simulink model "AbstractCombustionEngineCar_1_KHUSHI (3)"  (R2025a)
settings: Solver=FixedStepAuto  StartTime=0.0  StopTime=1200  FixedStep=0.001  MaxStep=0.001  RelTol=1e-3  AbsTol=1e-3
PreLoadFcn:
  | AbstractCombustionEngineCarSetup
libraries: fl_lib x18, nesl_utility x13, sdl_lib x5
CloseFcn:
  | try,close(h1_AbstractCombustionEngineCar),end
  | clear h1_AbstractCombustionEngineCar
  | 
  | try,close(h2_AbstractCombustionEngineCar),end
  | clear h2_AbstractCombustionEngineCar
  | 
  | try,close(h3_AbstractCombustionEngineCar),end
  | clear h3_AbstractCombustionEngineCar
  | 
  | clear tout_AbstractCombustionEngineCar
  | clear logsout_AbstractCombustionEngineCar
  | clear simlog_AbstractCombustionEngineCar
  | 
  | clear AbstractCombustionEngineCarInputplot
  | clear AbstractCombustionEngineCar_Signals
  | clear AbstractCombustionEngineCar_Bus
settings Model: Creator=The MathWorks, Inc.  LastModifiedBy=rajde
settings SolverCC: AutoScaleAbsTol=off  DaesscMode=Balanced  MaxZcPerStep=1.0
settings DataIOCC: SaveOutput=off  DSMLogging=off  ReturnWorkspaceOutputs=off  TimeSaveName=tout_AbstractCombustionEngineCar  SignalLoggingName=logsout_AbstractCombustionEngineCar  ReturnWorkspaceOutputsName=out_AbstractCombustionEngineCar
settings OptimizationCC: ReuseModelBlockBuffer=off
settings ModelReferenceCC: EnableRefExpFcnMdlSchedulingChecks=on
settings RTWCC: GPUComputeCapability=3.5
settings SimscapeCC: SimscapeLogType=all  SimscapeLogSimulationStatistics=on  SimscapeLogName=simlog_AbstractCombustionEngineCar  SimscapeLogLimitData=off

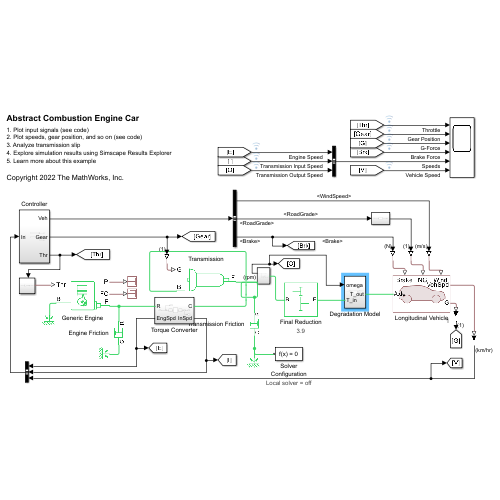
[thumbnail: Simulink's stored preview of the top-level diagram]
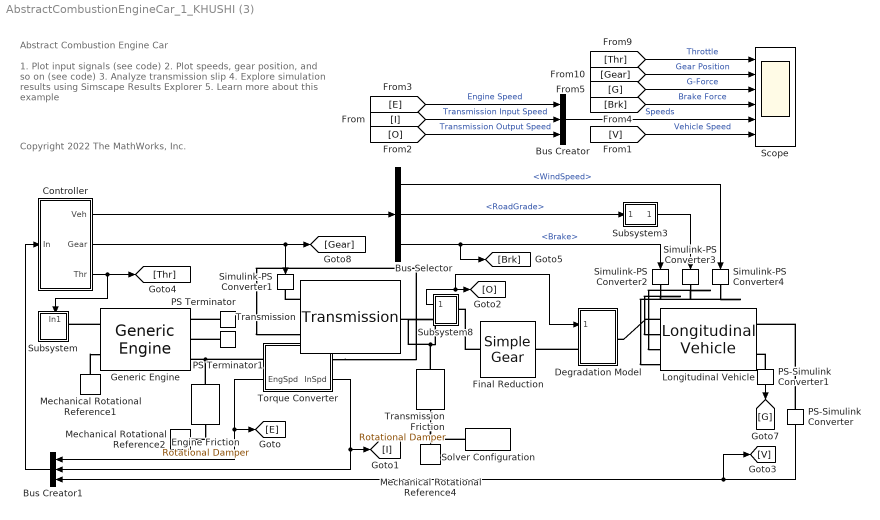
== system AbstractCombustionEngineCar_1_KHUSHI (3) ==
  note: 1. Plot input signals (see code)
      | 2. Plot speeds, gear position, and so on (see code)
      | 3. Analyze transmission slip
      | 4. Explore simulation results using Simscape Results Explorer
      | 5. Learn more about this example
  note: Abstract Combustion Engine Car
  note: Copyright 2022 The MathWorks, Inc.
  Bus Creator : BusCreator  Inputs=3
  Bus Creator1 : BusCreator  Inputs=3
  Bus Selector : BusSelector  OutputSignals=WindSpeed,RoadGrade,Brake
  Controller : Subsystem
  Degradation Model : Subsystem
  Engine Friction : fl_lib/Mechanical/Rotational Elements/Rotational Damper  D=0.01 N*m/rpm  w_specify=off  w_priority=None  w=0 rad/s  w_nominal_specify=off  w_nominal_value=1  w_nominal_unit=rad/s  t_specify=off  t_priority=None  t=0 N*m  t_nominal_specify=off  t_nominal_value=1  t_nominal_unit=N*m
  Final Reduction : sdl_lib/Gears/Simple Gear  ratio=3.9  rotation_direction=sdl.enum.shaftOutputDirection.same  friction_model=sdl.enum.gear_efficiencies_load.off  T_noload=0.1 N*m  T_nom=5 N*m  efficiency_nom=0.8  efficiency=0.8  temperature_TLU=[280, 300, 320] K  load_TLU=[1, 5, 10] N*m  efficiency_TLU=[.95, .9, .85]  efficiency_TLU2=[.85, .8, .75; .95, .9, .85; .85, .8, .7]  w_thr=0.01 rad/s  pwr_thr=0.001 W  enable_backlash=false  hardstop_model=simscape.enum.hardstop.smooth  backlash_distance=1e-3 mm  r_base=0.1 m  transition=1e-4 mm  backlash_stiffness=1e7 N/m  backlash_damping=1e6 N*s/m  coeff_rest=0  v_tol=0.001 m/s  f_tol=0 N  mu_visc=[0, 0] N*m*s/rad  thermal_mass=50 J/K  temperature_specify=off  temperature_priority=High  temperature=300 K  temperature_nominal_specify=off  temperature_nominal_value=1  temperature_nominal_unit=K  x_backlash_specify=off  x_backlash_priority=None  x_backlash=0 mm  x_backlash_nominal_specify=off  x_backlash_nominal_value=1  x_backlash_nominal_unit=mm  f_hardstop_specify=off  f_hardstop_priority=None  f_hardstop=0 N  f_hardstop_nominal_specify=off  f_hardstop_nominal_value=1  f_hardstop_nominal_unit=N  v_backlash_specify=off  v_backlash_priority=None  v_backlash=0 m/s  v_backlash_nominal_specify=off  v_backlash_nominal_value=1  v_backlash_nominal_unit=m/s
      settings: AttributesFormatString=%<ratio>
  Generic Engine : sdl_lib/Engines & Motors/Generic Engine  input_type=sdl.enum.GenericEngineInputType.NormalizedThrottle  model_parameterization=sdl.enum.engineParameterization.polynomial  engine_type=sdl.enum.engineType.SI  Trq_max=380 N*m  w_Trq_max=4300 rpm  P_max=150 kW  w_P_max=4500 rpm  w_max=6000 rpm  w_min=500 rpm  w_tab=[500, 1000, 2000, 3000, 4000, 5000, 6000, 7000] rpm  trq_tab=[380, 380, 380, 380, 350, 280, 200, 80] N*m  pwr_tab=[20, 40, 78, 120, 145, 148, 125, 60] kW  interp_method=simscape.enum.interpolation.linear  w_thr=100 rpm  model_inertia=sdl.enum.model_inertia.on  inertia=0.02 kg*m^2  initial_velocity=800 rpm  model_time_constant=sdl.enum.lagOffOn.off  time_constant=0.2 s  initial_normalized_throttle=0  fc_model=sdl.enum.fuel_consumption_model.FuelOff  fc_per_rev=25 mg/rev  fc_w_tab=[1000, 2000, 3000, 4000, 5000, 6000] rpm  fc_trq_tab=[0, 80, 160, 200, 240, 320, 360, 400] N*m  fc_tab=[.5, .9, 1.4, 1.6, 1.9, 2.7, 3.4, 4.4; 1, 1.7, 2.7, 3.1, 3.6, 5, 6, 7.4; 1.4, 2.7, 4, 4.8, 5.6, 7.5, 8.5, 10.5; 2, 3.6, 5.8, 6.7, 8, 10.4, 11.7, 13.3; 2.5, 4.8, 7.9, 9.4, 10.8, 14, 16.2, 18.6; 3.1, 6, 10.3, 11.9, 13.8, 18.4, 22, 26.5] g/s  bmep_tab=[0, 250, 500, 625, 750, 1000, 1150, 1250] kPa  bsfc_tab=[410, 380, 300, 280, 270, 290, 320, 380; 410, 370, 290, 270, 260, 270, 285, 320; 415, 380, 290, 275, 265, 270, 270, 300; 420, 390, 310, 290, 285, 280, 280, 285; 430, 410, 340, 320, 310, 300, 310, 320; 450, 430, 370, 340, 330, 330, 350, 380] g/(hr*kW)  fc_interp_method=simscape.enum.interpolation.linear  displaced_volume=400 cm^3  rev_per_cycle=2  idle_speed=simscape.enum.onoff.on  idle_speed_reference=800 rpm  tau_controller=0.1 s  idle_w_thr=10 rpm  redline=simscape.enum.onoff.off  redline_speed=7500 rpm  tau_redline=1 s  redline_w_thr=1 rpm
      settings: InternalSimscapePortConfiguration="{\"Bottom\":[],\"Left\":[{\"id\":\"ThrNorm\",\"label\":\"Thr\",\"type\":\"input\"},{\"id\":\"B\",\"label\":\"B\",\"type\":\"foundation.mechanical.rotational.rotational\"}],\"Right\":[{\"id\":\"P\",\"label\":\"P\",\"type\":\"output\"},{\"id\":\"FC\",\"label\":\"FC\",\"type\":\"output\"},{\"id\":\"F\",\"label\":\"F\",\"type\":\"foundation.mechanical.rotational.rotational\"}],\"Top\":[]}"
  Longitudinal Vehicle : sdl_lib/Tires & Vehicles/Longitudinal Vehicle  vehParamType=sdl.enum.VehicleParameterizationType.Large  M_vehicle=1200 kg  R_tireroll=0.3 m  C_tireroll=0.0136  C_airdrag=0.31  A_front=2.3 m^2  A_rl=120 N  B_rl=1.8 N*s/m  C_rl=0.389 N*s^2/m^2  g=9.81 m/s^2  V_1=0.3 m/s  w_1=0.01 rad/s  ShowBrakeIn=simscape.enum.onoff.on  ShowSlopeIn=simscape.enum.onoff.on  SlopeInputType=sdl.enum.VehicleLongitudinalRoadSlopeInputType.Grade  ShowWindIn=simscape.enum.onoff.on  ShowGOut=simscape.enum.onoff.on  air_density=1.184 kg/m^3  V_x_specify=off  V_x_priority=High  V_x=0 km/hr  V_x_nominal_specify=off  V_x_nominal_value=1  V_x_nominal_unit=m/s  trq_specify=off  trq_priority=None  trq=0 N*m  trq_nominal_specify=off  trq_nominal_value=1  trq_nominal_unit=N*m  w_specify=off  w_priority=None  w=0 rad/s  w_nominal_specify=off  w_nominal_value=1  w_nominal_unit=rad/s
      settings: InternalSimscapePortConfiguration="{\"Bottom\":[],\"Left\":[{\"id\":\"Axle\",\"label\":\"Axle\",\"type\":\"foundation.mechanical.rotational.rotational\"}],\"Right\":[{\"id\":\"v_out\",\"label\":\"VehSpd\",\"type\":\"output\"},{\"id\":\"G_out\",\"label\":\"G\",\"type\":\"output\"}],\"Top\":[{\"id\":\"brkF\",\"label\":\"Brake\",\"type\":\"input\"},{\"id\":\"grade_norm\",\"label\":\"NG\",\"type\":\"input\"},{\"id\":\"V_wind\",\"label\":\"Wind\",\"type\":\"input\"}]}"
  Mechanical Rotational Reference1 : fl_lib/Mechanical/Rotational Elements/Mechanical Rotational Reference
  Mechanical Rotational Reference2 : fl_lib/Mechanical/Rotational Elements/Mechanical Rotational Reference
  Mechanical Rotational Reference4 : fl_lib/Mechanical/Rotational Elements/Mechanical Rotational Reference
  PS Terminator : fl_lib/Physical Signals/Sinks/PS Terminator
  PS Terminator1 : fl_lib/Physical Signals/Sinks/PS Terminator
  PS-Simulink Converter : nesl_utility/PS-Simulink Converter  PhysicalDomain=network_engine_domain  SubClassName=ps_output  LeftPortType=input  RightPortType=output  PseudoPeriodic=off  Frequencies=[]  VectorFormat=inherit  Unit=km/hr  AffineConversion=off
  PS-Simulink Converter1 : nesl_utility/PS-Simulink Converter  PhysicalDomain=network_engine_domain  SubClassName=ps_output  LeftPortType=input  RightPortType=output  PseudoPeriodic=off  Frequencies=[]  VectorFormat=inherit  Unit=1  AffineConversion=off
  Scope : Scope  NumInputPorts=6
      settings: ActiveDisplayYMinimum=-11.25  ActiveDisplayYMaximum=101.25
  Simulink-PS Converter1 : nesl_utility/Simulink-PS Converter  PhysicalDomain=network_engine_domain  SubClassName=ps_input  LeftPortType=input  RightPortType=output  PseudoPeriodic=off  Frequencies=[]  NoiseDistribution=none  NoiseParameters=[]  Unit=1  AffineConversion=off  FilteringAndDerivatives=provide  SimscapeFilterOrder=1  InputFilterTimeConstant=0.001  UdotUserProvided=0
  Simulink-PS Converter2 : nesl_utility/Simulink-PS Converter  PhysicalDomain=network_engine_domain  SubClassName=ps_input  LeftPortType=input  RightPortType=output  PseudoPeriodic=off  Frequencies=[]  NoiseDistribution=none  NoiseParameters=[]  Unit=N  AffineConversion=off  FilteringAndDerivatives=provide  SimscapeFilterOrder=1  InputFilterTimeConstant=0.001  UdotUserProvided=0
  Simulink-PS Converter3 : nesl_utility/Simulink-PS Converter  PhysicalDomain=network_engine_domain  SubClassName=ps_input  LeftPortType=input  RightPortType=output  PseudoPeriodic=off  Frequencies=[]  NoiseDistribution=none  NoiseParameters=[]  Unit=1  AffineConversion=off  FilteringAndDerivatives=provide  SimscapeFilterOrder=1  InputFilterTimeConstant=0.001  UdotUserProvided=0
  Simulink-PS Converter4 : nesl_utility/Simulink-PS Converter  PhysicalDomain=network_engine_domain  SubClassName=ps_input  LeftPortType=input  RightPortType=output  PseudoPeriodic=off  Frequencies=[]  NoiseDistribution=none  NoiseParameters=[]  Unit=m/s  AffineConversion=off  FilteringAndDerivatives=provide  SimscapeFilterOrder=1  InputFilterTimeConstant=0.001  UdotUserProvided=0
  Solver Configuration : nesl_utility/Solver Configuration  PhysicalDomain=network_engine_domain  SubClassName=solver  LeftPortType=input  RightPortType=generic  Tones=[]  Harmonics=[]  SimulateNoise=off  Profile=off  UseLocalSampling=off  EnableSwitchedLinearOptims=on  FrequencyDomain=off  UseCCode=off  RelTol=0.001  AbsTol=0.001  MinStep=1e-09  ToWorkspace=off  RevertToSquareIcSolve=off  NumHomotopyIterations=100  PhasorMode=off  PhasorModeNumHarmonics=1  ConsistencySolver=NEWTON_XTOL_AFTER_FTOL  IndexReductionMethod=DerivativeReplacement  DoDC=off  ResidualTolerance=1e-09  ConsistencyTolSource=GLOBAL  ConsistencyAbsTol=0.001  ConsistencyRelTol=0.001  ConsistencyTolFactor=0.001  UseLocalSolver=off  LocalSolverChoice=NE_BACKWARD_EULER_ADVANCER  ResolveIndetEquations=on  FunctionEvalNumThread=1  LocalSolverSampleTime=0.001  DoFixedCost=off  MaxNonlinIter=3  MaxModeIter=2  ComputeImpulses=off  ImpulseIterations=2  LinearAlgebra=auto  LinearAlgebraNumThread=0  EquationFormulation=NE_TIME_EF  DelaysMemoryBudget=1024  AutomaticFiltering=on  FilteringTimeConstant=0.001  PartitionStorageMethod=AS_NEEDED  PartitionMemoryBudget=1024  PartitionMethod=ROBUST  MultibodyUseLocalSolver=off  MultibodyLocalSolverChoice=ODE1  MultibodyLocalSolverSampleTime=0.001
      settings: AttributesFormatString=Local solver = %<UseLocalSolver>
  Subsystem : Subsystem
      settings: PortSchema="{\"entries\":[{\"content\":{\"sides\":[{\"content\":{\"connectorIds\":[]},\"type\":\"ConnectorPlacement.EquallySpacedRectSide\",\"uuid\":\"38476285-4b1d-4cfe-b9ba-56388b6e142d\"},{\"content\":{\"connectorIds\":[\"RConn1\"],\"side\":\"RIGHT\"},\"type\":\"ConnectorPlacement.EquallySpacedRectSide\",\"uuid\":\"ba0e92dd-90b0-4ff2-bfbd-3d18e117ce00\"},{\"content\":{\"connectorIds\":[\"In1\"],\"side\":\"TOP\"},\"type\":\"ConnectorPlacement.EquallySpacedRectSide\",\"uuid\":\"d72bcda9-1129-409b-a624-7361223ab5f8\"}]},\"type\":\"ConnectorPlacement.EquallySpacedConnector\",\"uuid\":\"46949968-9b34-453f-a959-32b8a4fd4c57\"}],\"packageUris\":[\"http://schema.mathworks.com/mf0/Connector/R2020b\"],\"version\":\"1.0\"}"
  Subsystem3 : Subsystem
  Subsystem8 : Subsystem
      settings: PortSchema="{\"entries\":[{\"content\":{\"sides\":[{\"content\":{\"connectorIds\":[\"Out1\",\"LConn1\"]},\"type\":\"ConnectorPlacement.EquallySpacedRectSide\",\"uuid\":\"a87ce211-5ca3-4dba-a83b-da94e949f171\"},{\"content\":{\"connectorIds\":[\"RConn1\"],\"side\":\"RIGHT\"},\"type\":\"ConnectorPlacement.EquallySpacedRectSide\",\"uuid\":\"788867ba-271d-48ee-bf4b-70614e75db20\"},{\"content\":{\"connectorIds\":[],\"side\":\"TOP\"},\"type\":\"ConnectorPlacement.EquallySpacedRectSide\",\"uuid\":\"607020b5-dd3c-48e1-9492-c22d083697f7\"},{\"content\":{\"connectorIds\":[],\"side\":\"BOTTOM\"},\"type\":\"ConnectorPlacement.EquallySpacedRectSide\",\"uuid\":\"61462458-f4c7-4735-9817-1b1875f46976\"}]},\"type\":\"ConnectorPlacement.EquallySpacedConnector\",\"uuid\":\"473fa968-ffd5-4c8c-8204-df51e2cb909e\"}],\"packageUris\":[\"http://schema.mathworks.com/mf0/Connector/R2020b\"],\"version\":\"1.0\"}"
  Torque Converter : Subsystem
      settings: PortSchema="{\"entries\":[{\"content\":{\"sides\":[{\"content\":{\"connectorIds\":[\"LConn1\",\"Out2\"]},\"type\":\"ConnectorPlacement.EquallySpacedRectSide\",\"uuid\":\"617538e0-3440-487d-b133-1f4231421eb5\"},{\"content\":{\"connectorIds\":[\"RConn1\",\"Out1\"],\"side\":\"RIGHT\"},\"type\":\"ConnectorPlacement.EquallySpacedRectSide\",\"uuid\":\"0cc25c53-6bfd-4172-944f-9e7138ffc800\"},{\"content\":{\"connectorIds\":[],\"side\":\"TOP\"},\"type\":\"ConnectorPlacement.EquallySpacedRectSide\",\"uuid\":\"814870c3-fb4e-4999-b1ac-f0bc310280a4\"},{\"content\":{\"connectorIds\":[],\"side\":\"BOTTOM\"},\"type\":\"ConnectorPlacement.EquallySpacedRectSide\",\"uuid\":\"65ae3c81-05f8-4b99-bf66-538c9dc41f9a\"}]},\"type\":\"ConnectorPlacement.EquallySpacedConnector\",\"uuid\":\"f25e6ec4-4b55-4318-8ed3-0c35c2cb6893\"}],\"packageUris\":[\"http://schema.mathworks.com/mf0/Connector/R2020b\"],\"version\":\"1.0\"}"
  Transmission : sdl_lib/Gears/Transmission  gear_ratios=[2.3, 1.6, 1.2, 1, .8, .6]  reverse_ratio=-3  friction_model=sdl.enum.transmissionFriction.none  efficiency=0.95  efficiency_tlu=[.95, .95, .95, .95, .95, .95]  reverse_efficiency=0.90  pwr_thr=0.001 W  kp=3e5 N*m/rad  kv=3e4 N*m*s/rad  initial_torque=0 N*m  mu_visc=[0, 0] N*m*s/rad  t_friction=1000 N*m  t_locked=1000 N*m  shift_model=sdl.enum.transmissionShiftModel.instant  shift_time=200 ms  w_tol=0.001 rad/s  initial_state_locked=sdl.enum.initial_lock.locked  thermal_port=simscape.enum.thermaleffects.omit  thermal_mass=100 kJ/K  initial_temperature=300 K
      settings: InternalSimscapePortConfiguration="{\"Bottom\":[],\"Left\":[{\"id\":\"G\",\"label\":\"G\",\"type\":\"input\"},{\"id\":\"B\",\"label\":\"B\",\"type\":\"foundation.mechanical.rotational.rotational\"}],\"Right\":[{\"id\":\"F\",\"label\":\"F\",\"type\":\"foundation.mechanical.rotational.rotational\"}],\"Top\":[]}"
  Transmission Friction : fl_lib/Mechanical/Rotational Elements/Rotational Damper  D=0.001 N*m/rpm  w_specify=off  w_priority=None  w=0 rad/s  w_nominal_specify=off  w_nominal_value=1  w_nominal_unit=rad/s  t_specify=off  t_priority=None  t=0 N*m  t_nominal_specify=off  t_nominal_value=1  t_nominal_unit=N*m
  wires:
  Subsystem8/1(Spd) -> Degradation Model/1(omega), [O]
  [I] -> Bus Creator/2  "Transmission Input Speed"
  [O] -> Bus Creator/3  "Transmission Output Speed"
  [E] -> Bus Creator/1  "Engine Speed"
  Torque Converter/2(EngSpd) -> [E], Bus Creator1/1
  PS-Simulink Converter/1 -> Bus Creator1/3, [V]
  Bus Creator1/1 -> Controller/1(In)
  Controller/1(Veh) -> Bus Selector/1
  Torque Converter/1(InSpd) -> Bus Creator1/2, [I]
  [Thr] -> Scope/1  "Throttle"
  Bus Selector/3 -> [Brk], Simulink-PS Converter2/1  "<Brake>"
  Bus Selector/2 -> Subsystem3/1(In1)  "<RoadGrade>"
  Bus Selector/1 -> Simulink-PS Converter4/1  "<WindSpeed>"
  Subsystem3/1(Out1) -> Simulink-PS Converter3/1
  [V] -> Scope/6  "Vehicle Speed"
  Bus Creator/1 -> Scope/5  "Speeds"
  [G] -> Scope/3  "G-Force"
  Controller/3(Thr) -> [Thr], Subsystem/1(In1)
  Controller/2(Gear) -> Simulink-PS Converter1/1, [Gear]
  PS-Simulink Converter1/1 -> [G]
  [Brk] -> Scope/4  "Brake Force"
  [Gear] -> Scope/2  "Gear Position"
  connections:
  Torque Converter/LConn1 -- Engine Friction/LConn1 -- Generic Engine/RConn3
  Engine Friction/RConn1 -- Mechanical Rotational Reference2/LConn1
  Mechanical Rotational Reference1/LConn1 -- Generic Engine/LConn2
  Transmission Friction/LConn1 -- Transmission/RConn1 -- Subsystem8/LConn1
  Transmission/LConn1 -- Simulink-PS Converter1/RConn1
  Transmission Friction/RConn1 -- Solver Configuration/RConn1 -- Mechanical Rotational Reference4/LConn1
  PS-Simulink Converter/LConn1 -- Longitudinal Vehicle/RConn1
  Simulink-PS Converter3/RConn1 -- Longitudinal Vehicle/LConn3
  Simulink-PS Converter2/RConn1 -- Longitudinal Vehicle/LConn2
  Simulink-PS Converter4/RConn1 -- Longitudinal Vehicle/LConn4
  Torque Converter/RConn1 -- Transmission/LConn2
  Final Reduction/LConn1 -- Subsystem8/RConn1
  Generic Engine/LConn1 -- Subsystem/RConn1
  PS-Simulink Converter1/LConn1 -- Longitudinal Vehicle/RConn2
  PS Terminator/LConn1 -- Generic Engine/RConn1
  PS Terminator1/LConn1 -- Generic Engine/RConn2
  Degradation Model/LConn1 -- Final Reduction/RConn1
  Longitudinal Vehicle/LConn1 -- Degradation Model/RConn1

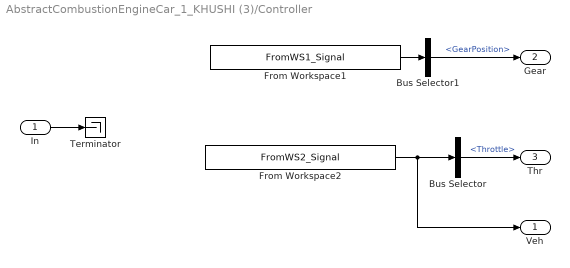
== system AbstractCombustionEngineCar_1_KHUSHI (3)/Controller ==
  In : Inport
  Bus Selector : BusSelector  OutputSignals=Throttle
  Bus Selector1 : BusSelector  OutputSignals=GearPosition
  From Workspace1 : FromWorkspace  VariableName=FromWS1_Signal  Interpolate=off  OutputAfterFinalValue=Holding final value
      settings: AttributesFormatString=Interpolate: %<Interpolate>
  From Workspace2 : FromWorkspace  VariableName=FromWS2_Signal  OutDataTypeStr=Bus: AbstractCombustionEngineCar_Bus  OutputAfterFinalValue=Holding final value
      settings: AttributesFormatString=Interpolate: %<Interpolate>
  Terminator : Terminator
  Veh : Outport
  Gear : Outport  Port=2
  Thr : Outport  Port=3
  wires:
  Bus Selector1/1 -> Gear/1  "<GearPosition>"
  From Workspace2/1 -> Veh/1, Bus Selector/1
  From Workspace1/1 -> Bus Selector1/1
  In/1 -> Terminator/1
  Bus Selector/1 -> Thr/1  "<Throttle>"

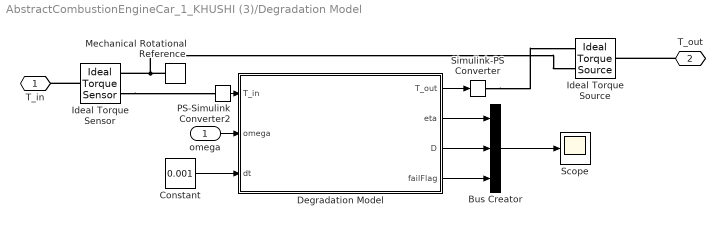
== system AbstractCombustionEngineCar_1_KHUSHI (3)/Degradation Model ==
  omega : Inport
  Bus Creator : BusCreator  Inputs=3
  Constant : Constant  Value=0.001
  Degradation Model : MATLAB Function  TreatAsAtomicUnit=on
  Ideal Torque Sensor : fl_lib/Mechanical/Mechanical Sensors/Ideal Torque Sensor
  Ideal Torque Source : fl_lib/Mechanical/Mechanical Sources/Ideal Torque Source
  Mechanical Rotational Reference : fl_lib/Mechanical/Rotational Elements/Mechanical Rotational Reference
  PS-Simulink Converter2 : nesl_utility/PS-Simulink Converter  PhysicalDomain=network_engine_domain  SubClassName=ps_output  LeftPortType=input  RightPortType=output  PseudoPeriodic=off  Frequencies=[]  VectorFormat=inherit  Unit=inherit  AffineConversion=off
  Scope : Scope
  Simulink-PS Converter : nesl_utility/Simulink-PS Converter  PhysicalDomain=network_engine_domain  SubClassName=ps_input  LeftPortType=input  RightPortType=output  PseudoPeriodic=off  Frequencies=[]  NoiseDistribution=none  NoiseParameters=[]  Unit=1  AffineConversion=off  FilteringAndDerivatives=provide  SimscapeFilterOrder=1  InputFilterTimeConstant=0.001  UdotUserProvided=0
  T_in : PMIOPort  Side=Left
  T_out : PMIOPort  Port=2  Side=Right
  wires:
  Constant/1 -> Degradation Model/3(dt)
  Degradation Model/2(eta) -> Bus Creator/1
  PS-Simulink Converter2/1 -> Degradation Model/1(T_in)
  Degradation Model/4(failFlag) -> Bus Creator/3
  Degradation Model/3(D) -> Bus Creator/2
  omega/1 -> Degradation Model/2(omega)
  Degradation Model/1(T_out) -> Simulink-PS Converter/1
  Bus Creator/1 -> Scope/1
  connections:
  Ideal Torque Sensor/LConn1 -- T_in/RConn1
  Ideal Torque Sensor/RConn2 -- PS-Simulink Converter2/LConn1
  Mechanical Rotational Reference/LConn1 -- Ideal Torque Source/RConn2 -- Ideal Torque Sensor/RConn1
  Simulink-PS Converter/RConn1 -- Ideal Torque Source/RConn1
  T_out/RConn1 -- Ideal Torque Source/LConn1

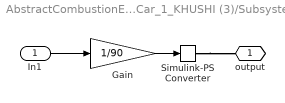
== system AbstractCombustionEngineCar_1_KHUSHI (3)/Subsystem ==
  In1 : Inport
  Gain : Gain  Gain=1/90
  Simulink-PS Converter : nesl_utility/Simulink-PS Converter  PhysicalDomain=network_engine_domain  SubClassName=ps_input  LeftPortType=input  RightPortType=output  PseudoPeriodic=off  Frequencies=[]  NoiseDistribution=none  NoiseParameters=[]  Unit=1  AffineConversion=off  FilteringAndDerivatives=provide  SimscapeFilterOrder=1  InputFilterTimeConstant=0.001  UdotUserProvided=0
  output : PMIOPort  Side=Right
  wires:
  Gain/1 -> Simulink-PS Converter/1
  In1/1 -> Gain/1
  connections:
  Simulink-PS Converter/RConn1 -- output/RConn1

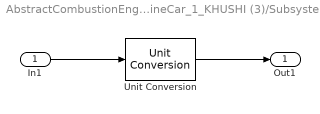
== system AbstractCombustionEngineCar_1_KHUSHI (3)/Subsystem3 ==
  In1 : Inport
  Unit Conversion : UnitConversion
  Out1 : Outport
  wires:
  In1/1 -> Unit Conversion/1
  Unit Conversion/1 -> Out1/1

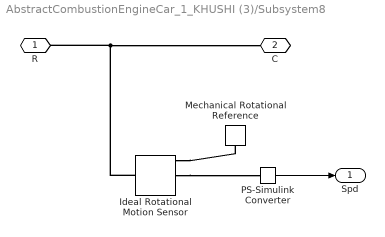
== system AbstractCombustionEngineCar_1_KHUSHI (3)/Subsystem8 ==
  Ideal Rotational Motion Sensor : fl_lib/Mechanical/Mechanical Sensors/Ideal Rotational Motion Sensor  reference=foundation.enum.MeasurementReference.difference  acceleration_port=false  velocity_port=true  position_port=true  wrap_angle=simscape.enum.onoff.off  offset=0 rad
  Mechanical Rotational Reference : fl_lib/Mechanical/Rotational Elements/Mechanical Rotational Reference
  PS-Simulink Converter : nesl_utility/PS-Simulink Converter  PhysicalDomain=network_engine_domain  SubClassName=ps_output  LeftPortType=input  RightPortType=output  PseudoPeriodic=off  Frequencies=[]  VectorFormat=inherit  Unit=rpm  AffineConversion=off
  R : PMIOPort  Side=Left
  C : PMIOPort  Port=2  Side=Right
  Spd : Outport  Unit=rpm
  wires:
  PS-Simulink Converter/1 -> Spd/1
  connections:
  Ideal Rotational Motion Sensor/RConn2 -- PS-Simulink Converter/LConn1
  Ideal Rotational Motion Sensor/RConn1 -- Mechanical Rotational Reference/LConn1
  Ideal Rotational Motion Sensor/LConn1 -- C/RConn1 -- R/RConn1

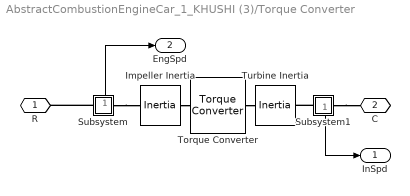
== system AbstractCombustionEngineCar_1_KHUSHI (3)/Torque Converter ==
  Impeller Inertia : fl_lib/Mechanical/Rotational Elements/Inertia  inertia=0.01 kg*m^2  num_ports=foundation.enum.numPorts2.two  w_specify=on  w_priority=None  w=0 rad/s  w_nominal_specify=off  w_nominal_value=1  w_nominal_unit=rad/s  t_specify=off  t_priority=None  t=0 N*m  t_nominal_specify=off  t_nominal_value=1  t_nominal_unit=N*m
      settings: InternalSimscapePortConfiguration="{\"Bottom\":[],\"Left\":[{\"id\":\"I\",\"label\":\"\",\"type\":\"foundation.mechanical.rotational.rotational\"}],\"Right\":[{\"id\":\"J\",\"label\":\"\",\"type\":\"foundation.mechanical.rotational.rotational\"}],\"Top\":[]}"
  Subsystem : Subsystem
      settings: PortSchema="{\"entries\":[{\"content\":{\"sides\":[{\"content\":{\"connectorIds\":[\"LConn1\"]},\"type\":\"ConnectorPlacement.EquallySpacedRectSide\",\"uuid\":\"a87ce211-5ca3-4dba-a83b-da94e949f171\"},{\"content\":{\"connectorIds\":[\"RConn1\"],\"side\":\"RIGHT\"},\"type\":\"ConnectorPlacement.EquallySpacedRectSide\",\"uuid\":\"788867ba-271d-48ee-bf4b-70614e75db20\"},{\"content\":{\"connectorIds\":[\"Out1\"],\"side\":\"TOP\"},\"type\":\"ConnectorPlacement.EquallySpacedRectSide\",\"uuid\":\"607020b5-dd3c-48e1-9492-c22d083697f7\"}]},\"type\":\"ConnectorPlacement.EquallySpacedConnector\",\"uuid\":\"473fa968-ffd5-4c8c-8204-df51e2cb909e\"}],\"packageUris\":[\"http://schema.mathworks.com/mf0/Connector/R2020b\"],\"version\":\"1.0\"}"
  Subsystem1 : Subsystem
      settings: PortSchema="{\"entries\":[{\"content\":{\"sides\":[{\"content\":{\"connectorIds\":[\"LConn1\"]},\"type\":\"ConnectorPlacement.EquallySpacedRectSide\",\"uuid\":\"a87ce211-5ca3-4dba-a83b-da94e949f171\"},{\"content\":{\"connectorIds\":[\"RConn1\"],\"side\":\"RIGHT\"},\"type\":\"ConnectorPlacement.EquallySpacedRectSide\",\"uuid\":\"788867ba-271d-48ee-bf4b-70614e75db20\"},{\"content\":{\"connectorIds\":[],\"side\":\"TOP\"},\"type\":\"ConnectorPlacement.EquallySpacedRectSide\",\"uuid\":\"607020b5-dd3c-48e1-9492-c22d083697f7\"},{\"content\":{\"connectorIds\":[\"Out1\"],\"side\":\"BOTTOM\"},\"type\":\"ConnectorPlacement.EquallySpacedRectSide\",\"uuid\":\"80162497-1058-420d-8454-863f1e6cbabb\"}]},\"type\":\"ConnectorPlacement.EquallySpacedConnector\",\"uuid\":\"473fa968-ffd5-4c8c-8204-df51e2cb909e\"}],\"packageUris\":[\"http://schema.mathworks.com/mf0/Connector/R2020b\"],\"version\":\"1.0\"}"
  Torque Converter : sdl_lib/Couplings & Drives/Torque Converter  coast_mode_modeling=sdl.enum.torqueConverterContinuousTwomode.twomode  SR_drive_tlu=[0, .5, .6, .7, .8, .87, .92, .94, .96, .97, 1]  TR_drive_tlu=[2.232, 1.5462, 1.4058, 1.2746, 1.1528, 1.0732, 1.0192, 1, 1, 1, 1]  CF_drive_tlu=1e-4 * [.72558, .66322, .63463, .59042, .51331, .4144, .29287, .22444, .12186, .04386, 0] N*m/rpm^2  SR_coast_tlu=[0, .5, .6, .7, .8, .87, .92, .94, .96, .97, 1]  CF_coast_tlu=1e-4 * [.5079, .4643, .4442, .4133, .3593, .2901, .205, .1571, .0853, .0307, 0] N*m/rpm^2  iniMode=sdl.enum.torqueConverterInitialMode.drive  delta_w=1 rpm  n_vector=[0, .5, .6, .7, .8, .87, .92, .94, .96, .97]  trq_vector=[2.232, 1.5462, 1.4058, 1.2746, 1.1528, 1.0732, 1.0192, .9983, .9983, .9983]  cf_vector_parameterization=sdl.enum.torqueConverterCFParameterization.SpeedToSqrtTorque  cf_vector_reference_speed=sdl.enum.torqueConverterCFReferenceSpeed.ImpellerSpeedAlways  cf_vector=[12.2938, 12.8588, 13.1452, 13.6285, 14.6163, 16.2675, 19.3503, 22.1046, 29.9986, 50] rad/(N^(1/2)*m^(1/2)*s)  cf_vector_sq=1e-3 * [6.616, 6.048, 5.787, 5.384, 4.681, 3.779, 2.671, 2.047, 1.111, .4] N*m*s^2/rad^2  interp_method=simscape.enum.interpolation.linear  extrap_method=simscape.enum.extrapolation.linear  model_lag=sdl.enum.torqueConverterLagOnOff.LagOff  tau=.02 s  initial_trq_ratio=0
      settings: InternalSimscapePortConfiguration="{\"Bottom\":[],\"Left\":[{\"id\":\"I\",\"label\":\"I\",\"type\":\"foundation.mechanical.rotational.rotational\"}],\"Right\":[{\"id\":\"T\",\"label\":\"T\",\"type\":\"foundation.mechanical.rotational.rotational\"}],\"Top\":[]}"
  Turbine Inertia : fl_lib/Mechanical/Rotational Elements/Inertia  inertia=0.01 kg*m^2  num_ports=foundation.enum.numPorts2.two  w_specify=on  w_priority=None  w=0 rad/s  w_nominal_specify=off  w_nominal_value=1  w_nominal_unit=rad/s  t_specify=off  t_priority=None  t=0 N*m  t_nominal_specify=off  t_nominal_value=1  t_nominal_unit=N*m
      settings: InternalSimscapePortConfiguration="{\"Bottom\":[],\"Left\":[{\"id\":\"I\",\"label\":\"\",\"type\":\"foundation.mechanical.rotational.rotational\"}],\"Right\":[{\"id\":\"J\",\"label\":\"\",\"type\":\"foundation.mechanical.rotational.rotational\"}],\"Top\":[]}"
  R : PMIOPort  Side=Left
  C : PMIOPort  Port=2  Side=Right
  InSpd : Outport
  EngSpd : Outport  Port=2
  wires:
  Subsystem/1(Spd) -> EngSpd/1
  Subsystem1/1(Spd) -> InSpd/1
  connections:
  Torque Converter/RConn1 -- Turbine Inertia/RConn1
  Subsystem/LConn1 -- R/RConn1
  Subsystem1/LConn1 -- Turbine Inertia/LConn1
  Impeller Inertia/LConn1 -- Torque Converter/LConn1
  Subsystem/RConn1 -- Impeller Inertia/RConn1
  Subsystem1/RConn1 -- C/RConn1

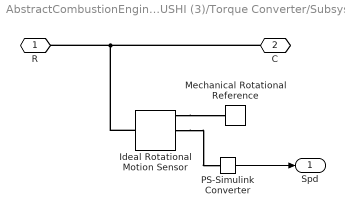
== system AbstractCombustionEngineCar_1_KHUSHI (3)/Torque Converter/Subsystem ==
  Ideal Rotational Motion Sensor : fl_lib/Mechanical/Mechanical Sensors/Ideal Rotational Motion Sensor  reference=foundation.enum.MeasurementReference.difference  acceleration_port=false  velocity_port=true  position_port=true  wrap_angle=simscape.enum.onoff.off  offset=0 rad
  Mechanical Rotational Reference : fl_lib/Mechanical/Rotational Elements/Mechanical Rotational Reference
  PS-Simulink Converter : nesl_utility/PS-Simulink Converter  PhysicalDomain=network_engine_domain  SubClassName=ps_output  LeftPortType=input  RightPortType=output  PseudoPeriodic=off  Frequencies=[]  VectorFormat=inherit  Unit=rpm  AffineConversion=off
  R : PMIOPort  Side=Left
  C : PMIOPort  Port=2  Side=Right
  Spd : Outport  Unit=rpm
  wires:
  PS-Simulink Converter/1 -> Spd/1
  connections:
  Ideal Rotational Motion Sensor/RConn2 -- PS-Simulink Converter/LConn1
  Ideal Rotational Motion Sensor/LConn1 -- C/RConn1 -- R/RConn1
  Ideal Rotational Motion Sensor/RConn1 -- Mechanical Rotational Reference/LConn1

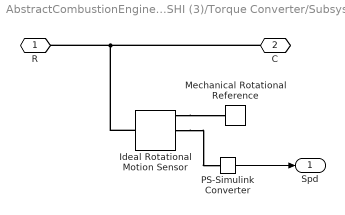
== system AbstractCombustionEngineCar_1_KHUSHI (3)/Torque Converter/Subsystem1 ==
  Ideal Rotational Motion Sensor : fl_lib/Mechanical/Mechanical Sensors/Ideal Rotational Motion Sensor  reference=foundation.enum.MeasurementReference.difference  acceleration_port=false  velocity_port=true  position_port=true  wrap_angle=simscape.enum.onoff.off  offset=0 rad
  Mechanical Rotational Reference : fl_lib/Mechanical/Rotational Elements/Mechanical Rotational Reference
  PS-Simulink Converter : nesl_utility/PS-Simulink Converter  PhysicalDomain=network_engine_domain  SubClassName=ps_output  LeftPortType=input  RightPortType=output  PseudoPeriodic=off  Frequencies=[]  VectorFormat=inherit  Unit=rpm  AffineConversion=off
  R : PMIOPort  Side=Left
  C : PMIOPort  Port=2  Side=Right
  Spd : Outport  Unit=rpm
  wires:
  PS-Simulink Converter/1 -> Spd/1
  connections:
  Ideal Rotational Motion Sensor/RConn2 -- PS-Simulink Converter/LConn1
  Ideal Rotational Motion Sensor/LConn1 -- C/RConn1 -- R/RConn1
  Ideal Rotational Motion Sensor/RConn1 -- Mechanical Rotational Reference/LConn1

== matlab function AbstractCombustionEngineCar_1_KHUSHI (3)/Degradation Model/Degradation Model ==
  data: T_in input; T_out output; omega input; dt input; eta output; D output; failFlag output
function [T_out, eta, D, failFlag] = DegradationModel(T_in, omega, dt)
% Inputs:
%   T_in  - Input torque [Nm]
%   omega - Shaft speed [rad/s]
%   dt    - Time step [s]

% Outputs:
%   T_out    - Degraded output torque [Nm]
%   eta      - Instantaneous efficiency [0–1]
%   D        - Cumulative damage (0–1)
%   failFlag - 1 if failure reached, else 0


persistent D_prev eta_prev initialized
if isempty(initialized)
    D_prev = 0;      % initial degradation
    eta_prev = 0.96; % initial efficiency (assumed)
    initialized = true;
end

%Assumed Parameters(tune as per your req)
eta0     = 0.96;      % initial efficiency
Dfail    = 1.0;       % failure threshold
etaCrit  = 0.8 * eta0; % critical efficiency threshold
gamma    = 2;         % drop rate
k1       = 1e-8;      % torque-cycle degradation coeff
p        = 2;         % torque exponent
k2       = 5e-6;      % time-based wear coeff
k3       = 1e-10;     % friction wear coeff

%degradation rates
dD_cycle    = k1 * abs(T_in)^p * dt;                     % fatigue wear
dD_time     = k2 * dt;                                   % time-based
dD_friction = k3 * abs(T_in * omega) * (1 - eta_prev) * dt; % friction wear

%cumulative damage
D = D_prev + dD_cycle + dD_time + dD_friction;
D = min(D, Dfail);

% damage to efficiency
eta = eta0 * (1 - (D / Dfail)^gamma);
eta = max(0, eta);

%degradaed torque
T_out = T_in * eta;

%stop in case of failure
if (D >= Dfail) || (eta <= etaCrit)
    failFlag = 1;
else
    failFlag = 0;
end

%store states
D_prev = D;
eta_prev = eta;
